simulink subsystem "HVACEmpiricalRef"  (R2024b)
settings: Solver=VariableStepAuto  StartTime=0.0  StopTime=10.0  RelTol=1e-3
undefined symbols (not defined in the file or in its folder): HVAC, vehicleThermal
libraries: fl_lib x70, nesl_utility x25, ee_lib x1
(part 1 of 2)
Description:
  | HVAC Empirical Reference
  | 
  | ⚡ Main Features:
  | - Empirical-based HVAC model with cabin and refrigeration subsystems
  | - Inputs: environment temperature, blower, PTC, compressor commands
  | - Refrigeration block models evaporator and compressor operation
  | - PTC heater and blower for cabin heating and airflow control
  | - Controlled current source represents HVAC electrical power draw
  | - Energy block tracks HVAC consumption from HV bus
  | 
  | 📤 Outputs: Cabin Temperature, HVAC Energy, Blower/Cooler/PTC States
  | 
  | 📌 Use Case: Fast empirical HVAC representation for cabin comfort and energy demand studies
settings Model: Creator=shachind  LastModifiedBy=jjha
settings RTWCC: GPUComputeCapability=3.5

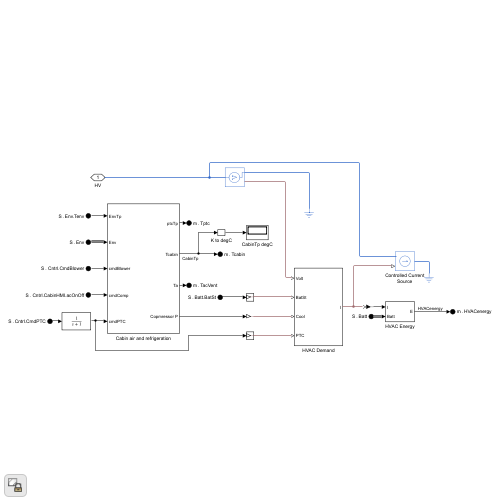
[thumbnail: Simulink's stored preview of the top-level diagram]
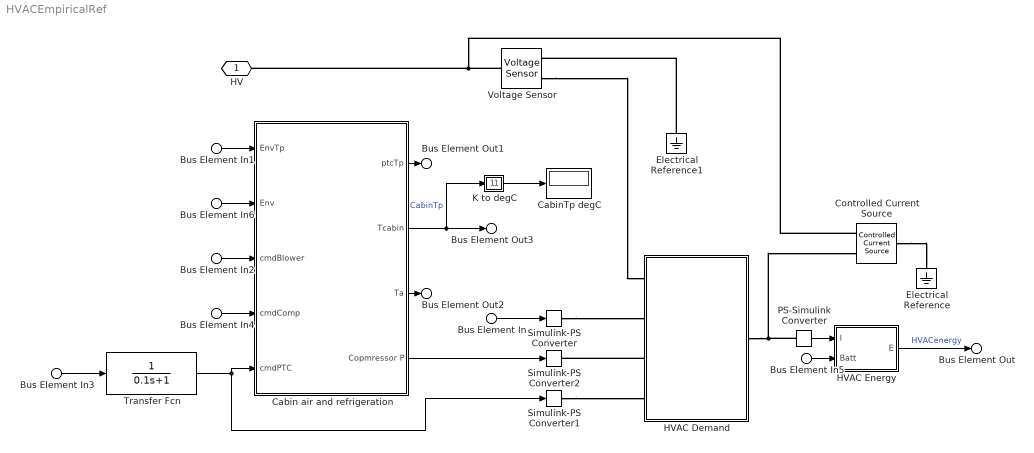
== system HVACEmpiricalRef ==
  Bus Element In5 : Inport  PortName=S  Element=Batt
  Bus Element In : Inport  PortName=S  Element=Batt.BatSt
  Bus Element In2 : Inport  PortName=S  Element=Cntrl.CmdBlower
  Bus Element In3 : Inport  PortName=S  Element=Cntrl.CmdPTC
  Bus Element In4 : Inport  PortName=S  Element=Cntrl.acOnOff
  Bus Element In6 : Inport  PortName=S  Element=Env
  Bus Element In1 : Inport  PortName=S  Element=Env.Tenv
  Cabin air and refrigeration : Subsystem
  CabinTp degC : Display
  Controlled Current Source : fl_lib/Electrical/Electrical Sources/Controlled Current Source
  Electrical Reference : fl_lib/Electrical/Electrical Elements/Electrical Reference
  Electrical Reference1 : fl_lib/Electrical/Electrical Elements/Electrical Reference
  HVAC Demand : Subsystem
  HVAC Energy : Subsystem
  K to degC : Subsystem
  PS-Simulink Converter : nesl_utility/PS-Simulink Converter  PhysicalDomain=network_engine_domain  SubClassName=ps_output  LeftPortType=input  RightPortType=output  PseudoPeriodic=off  Frequencies=[]  VectorFormat=inherit  Unit=inherit  AffineConversion=off
  Simulink-PS Converter : nesl_utility/Simulink-PS Converter  PhysicalDomain=network_engine_domain  SubClassName=ps_input  LeftPortType=input  RightPortType=output  PseudoPeriodic=off  Frequencies=[]  NoiseDistribution=none  NoiseParameters=[]  Unit=1  AffineConversion=off  FilteringAndDerivatives=provide  SimscapeFilterOrder=1  InputFilterTimeConstant=0.001  UdotUserProvided=0
  Simulink-PS Converter1 : nesl_utility/Simulink-PS Converter  PhysicalDomain=network_engine_domain  SubClassName=ps_input  LeftPortType=input  RightPortType=output  PseudoPeriodic=off  Frequencies=[]  NoiseDistribution=none  NoiseParameters=[]  Unit=W  AffineConversion=off  FilteringAndDerivatives=provide  SimscapeFilterOrder=1  InputFilterTimeConstant=0.001  UdotUserProvided=0
  Simulink-PS Converter2 : nesl_utility/Simulink-PS Converter  PhysicalDomain=network_engine_domain  SubClassName=ps_input  LeftPortType=input  RightPortType=output  PseudoPeriodic=off  Frequencies=[]  NoiseDistribution=none  NoiseParameters=[]  Unit=W  AffineConversion=off  FilteringAndDerivatives=provide  SimscapeFilterOrder=1  InputFilterTimeConstant=0.001  UdotUserProvided=0
  Transfer Fcn : TransferFcn  Denominator=[0.1 1]
  Voltage Sensor : fl_lib/Electrical/Electrical Sensors/Voltage Sensor
  HV : PMIOPort  Side=Left
  Bus Element Out : Outport  PortName=m  Element=HVACenergy
  Bus Element Out1 : Outport  PortName=m  Element=Tptc
  Bus Element Out3 : Outport  PortName=m  Element=Tcabin
  Bus Element Out2 : Outport  PortName=m  Element=TacVent
  wires:
  Bus Element In6/1 -> Cabin air and refrigeration/2(Env)
  Bus Element In2/1 -> Cabin air and refrigeration/3(cmdBlower)
  Cabin air and refrigeration/1(ptcTp) -> Bus Element Out1/1
  HVAC Energy/1(E) -> Bus Element Out/1  "HVACenergy"
  Bus Element In1/1 -> Cabin air and refrigeration/1(EnvTp)
  PS-Simulink Converter/1 -> HVAC Energy/1(I)
  Bus Element In5/1 -> HVAC Energy/2(Batt)
  Cabin air and refrigeration/4(Copmressor P) -> Simulink-PS Converter2/1
  Bus Element In3/1 -> Transfer Fcn/1
  Bus Element In/1 -> Simulink-PS Converter/1
  Cabin air and refrigeration/3(Ta) -> Bus Element Out2/1
  Bus Element In4/1 -> Cabin air and refrigeration/4(cmdComp)
  K to degC/1("  ") -> CabinTp degC/1
  Cabin air and refrigeration/2(Tcabin) -> K to degC/1(" "), Bus Element Out3/1  "CabinTp"
  Transfer Fcn/1 -> Simulink-PS Converter1/1, Cabin air and refrigeration/5(cmdPTC)
  connections:
  Controlled Current Source/RConn2 -- HV/RConn1 -- Voltage Sensor/LConn1
  PS-Simulink Converter/LConn1 -- Controlled Current Source/RConn1 -- HVAC Demand/RConn1
  Controlled Current Source/LConn1 -- Electrical Reference/LConn1
  Voltage Sensor/RConn1 -- HVAC Demand/LConn1
  Simulink-PS Converter/RConn1 -- HVAC Demand/LConn2
  HVAC Demand/LConn3 -- Simulink-PS Converter2/RConn1
  Simulink-PS Converter1/RConn1 -- HVAC Demand/LConn4
  Electrical Reference1/LConn1 -- Voltage Sensor/RConn2

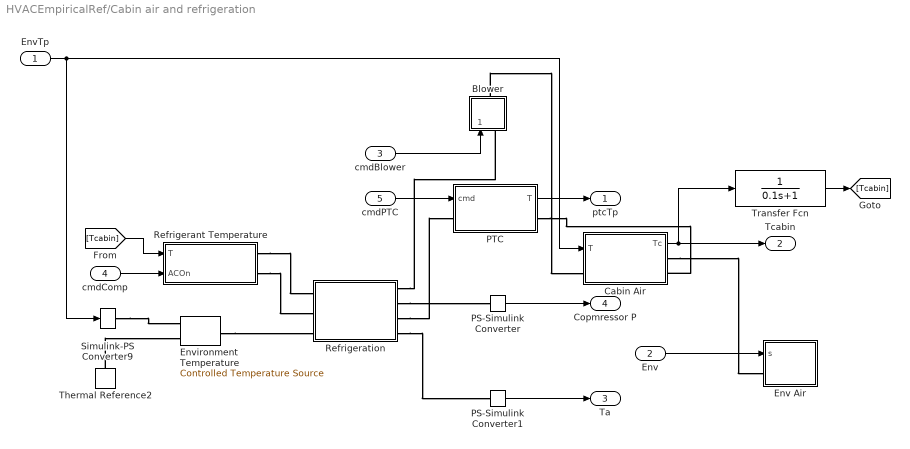
== system HVACEmpiricalRef/Cabin air and refrigeration ==
  EnvTp : Inport
  Env : Inport  Port=2
  cmdBlower : Inport  Port=3
  cmdComp : Inport  Port=4
  cmdPTC : Inport  Port=5
  Blower : Subsystem  Tag=PublishSubsystem
      mask Display:
      | plot(100*cos(linspace(0, 2*pi, 500)), 100*sin(linspace(0, 2*pi, 500)))
      | plot([28 80], [96 -60])
      | plot([-28 -80], [96 -60])
      | patch(-50*sin(3*linspace(0, pi, 500)).*cos(linspace(0, pi, 500)), -50*sin(3*linspace(0, pi, 500)).*sin(linspace(0, pi, 500)), [0 0 0])
  Cabin Air : Subsystem
      mask Display: disp(get_param(gcb, 'Name'))
  Env Air : Subsystem
  Environment Temperature : fl_lib/Thermal/Thermal Sources/Controlled Temperature Source
  PS-Simulink Converter : nesl_utility/PS-Simulink Converter  PhysicalDomain=network_engine_domain  SubClassName=ps_output  LeftPortType=input  RightPortType=output  PseudoPeriodic=off  Frequencies=[]  VectorFormat=inherit  Unit=inherit  AffineConversion=off
  PS-Simulink Converter1 : nesl_utility/PS-Simulink Converter  PhysicalDomain=network_engine_domain  SubClassName=ps_output  LeftPortType=input  RightPortType=output  PseudoPeriodic=off  Frequencies=[]  VectorFormat=inherit  Unit=inherit  AffineConversion=off
  PTC : Subsystem
      mask Display: disp(get_param(gcb, 'Name'))
  Refrigerant Temperature : Subsystem  mask{RefTemp=225.25}
      mask prompts: RefTemp "Condensor Refrigerant Temperature  [K]"
      mask DialogControl Refrigerant_temp Prompt: Parameters
  Refrigeration : Subsystem  mask{mRefEvap=1, mTubeEvap=1, tubeDiaEvap=0.01, tubeThickEvap=0.001, tubeLEvap=10, htcBoil=400, mRefCond=1, tubeDiaCond=0.01, tubeThickCond=0.001, tubeLCond=10, htcCondense=400, systemEfficiency=0.75}
      mask prompts: mRefEvap "Refrigerant mass inside evaporator (kg)"; mTubeEvap "Tube mass (kg)"; tubeDiaEvap "Tube outer diameter (m)"; tubeThickEvap "Tube wall thickness (m)"; tubeLEvap "Total length of the tube (m)"; htcBoil "Nucleate boiling HTC (W/K-m^2)"; mRefCond "Refrigerant mass inside Condensor (kg)"; tubeDiaCond "Tube outer diameter (m)"; tubeThickCond "Tube wall thickness (m)"; tubeLCond "Total length of the tube (m)"; htcCondense "Film condensation HTC (W/K-m^2)"; systemEfficiency "Overall system efficiency"
      mask DialogControl Container2 Prompt: Evaporator params
      mask DialogControl Container3 Prompt: Condensor params
      mask DialogControl Container4 Prompt: System params
      mask Display: disp(get_param(gcb, 'Name'))
  Simulink-PS Converter9 : nesl_utility/Simulink-PS Converter  PhysicalDomain=network_engine_domain  SubClassName=ps_input  LeftPortType=input  RightPortType=output  PseudoPeriodic=off  Frequencies=[]  NoiseDistribution=none  NoiseParameters=[]  Unit=K  AffineConversion=on  FilteringAndDerivatives=provide  SimscapeFilterOrder=1  InputFilterTimeConstant=0.001  UdotUserProvided=0
  Thermal Reference2 : fl_lib/Thermal/Thermal Elements/Thermal Reference
  Transfer Fcn : TransferFcn  Denominator=[0.1 1]
  ptcTp : Outport
  Tcabin : Outport  Port=2
  Ta : Outport  Port=3
  Copmressor P : Outport  Port=4
  wires:
  Transfer Fcn/1 -> [Tcabin]
  Env/1 -> Env Air/1(s)
  Cabin Air/1(Tc) -> Tcabin/1, Transfer Fcn/1
  PS-Simulink Converter1/1 -> Ta/1
  PS-Simulink Converter/1 -> Copmressor P/1
  PTC/1(T) -> ptcTp/1
  cmdBlower/1 -> Blower/1(cmd_blower)
  [Tcabin] -> Refrigerant Temperature/1(T)
  EnvTp/1 -> Simulink-PS Converter9/1, Cabin Air/1(T)
  cmdComp/1 -> Refrigerant Temperature/2(ACOn)
  cmdPTC/1 -> PTC/1(cmd)
  connections:
  Cabin Air/RConn1 -- Env Air/LConn1
  PTC/RConn1 -- Cabin Air/RConn2
  Blower/RConn1 -- Cabin Air/LConn1
  Refrigeration/RConn4 -- PS-Simulink Converter1/LConn1
  Refrigeration/RConn3 -- PTC/LConn1
  Refrigeration/RConn2 -- PS-Simulink Converter/LConn1
  Refrigeration/RConn1 -- Blower/LConn1
  Simulink-PS Converter9/RConn1 -- Environment Temperature/RConn1
  Environment Temperature/LConn1 -- Refrigeration/LConn3
  Thermal Reference2/LConn1 -- Environment Temperature/RConn2
  Refrigerant Temperature/RConn2 -- Refrigeration/LConn2
  Refrigerant Temperature/RConn1 -- Refrigeration/LConn1

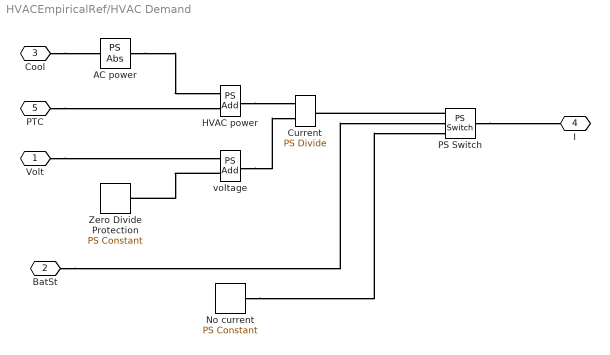
== system HVACEmpiricalRef/HVAC Demand ==
  AC power : fl_lib/Physical Signals/Nonlinear Operators/PS Abs
      settings: InternalSimscapePortConfiguration="{\"Bottom\":[],\"Left\":[{\"id\":\"I\",\"label\":\"\",\"type\":\"input\"}],\"Right\":[{\"id\":\"O\",\"label\":\"\",\"type\":\"output\"}],\"Top\":[]}"
  "Current " : fl_lib/Physical Signals/Functions/PS Divide
  HVAC power : fl_lib/Physical Signals/Functions/PS Add
  No current : fl_lib/Physical Signals/Sources/PS Constant  constant=0 A
  PS Switch : fl_lib/Physical Signals/Nonlinear Operators/PS Switch  Threshold=0.5
      settings: InternalSimscapePortConfiguration="{\"Bottom\":[],\"Left\":[{\"id\":\"I1\",\"label\":\"\",\"type\":\"input\"},{\"id\":\"I2\",\"label\":\"\",\"type\":\"input\"},{\"id\":\"I3\",\"label\":\"\",\"type\":\"input\"}],\"Right\":[{\"id\":\"O\",\"label\":\"\",\"type\":\"output\"}],\"Top\":[]}"
  Zero Divide Protection : fl_lib/Physical Signals/Sources/PS Constant  constant=10 V
  voltage : fl_lib/Physical Signals/Functions/PS Add
  Volt : PMIOPort  Side=Left
  BatSt : PMIOPort  Port=2  Side=Left
  Cool : PMIOPort  Port=3  Side=Left
  I : PMIOPort  Port=4  Side=Right
  PTC : PMIOPort  Port=5  Side=Left
  connections:
  Volt/RConn1 -- voltage/LConn1
  HVAC power/RConn1 -- "Current "/LConn1
  PTC/RConn1 -- HVAC power/LConn2
  Cool/RConn1 -- AC power/LConn1
  AC power/RConn1 -- HVAC power/LConn1
  voltage/LConn2 -- Zero Divide Protection/RConn1
  voltage/RConn1 -- "Current "/LConn2
  PS Switch/RConn1 -- I/RConn1
  BatSt/RConn1 -- PS Switch/LConn2
  PS Switch/LConn1 -- "Current "/RConn1
  No current/RConn1 -- PS Switch/LConn3

== system HVACEmpiricalRef/HVAC Energy ==
  I : Inport
  Batt : Inport  Port=2
  Bus Selector : BusSelector  OutputSignals=BattSensor.BatVolt
  Constant : Constant  Value=3600
  Divide : Product  Inputs=*/
  Integrator : Integrator
  Product : Product
  E : Outport
  wires:
  Bus Selector/1 -> Product/2  "<BatVolt>"
  Product/1 -> Integrator/1
  Integrator/1 -> Divide/1
  Constant/1 -> Divide/2
  Batt/1 -> Bus Selector/1
  Divide/1 -> E/1
  I/1 -> Product/1

== system HVACEmpiricalRef/K to degC ==
  " " : Inport
  Constant : Constant  Value=273.15
  Subtract : Sum  Inputs=+-
  "  " : Outport
  wires:
  Constant/1 -> Subtract/2
  Subtract/1 -> "  "/1
  " "/1 -> Subtract/1

== system HVACEmpiricalRef/Cabin air and refrigeration/Blower ==
  cmd_blower : Inport
  Blower : fl_lib/Moist Air/Sources/Flow Rate Source (MA)  source_type=foundation.enum.constant_controlled.controlled  flow_type=foundation.enum.mass_volumetric_flow.volumetric  mass_flow=0 kg/s  volumetric_flow=0 m^3/s  volumetric_flow_conditions=foundation.enum.volumetric_flow_conditions.standard  p_std=0.101325 MPa  T_std=vehicleThermal.cabin_T_init K  RH_std=0.65  power_spec=foundation.enum.power_spec.isentropic  area_A=HVAC.cabin_duct_area m^2  area_B=HVAC.cabin_duct_area m^2
      settings: InternalSimscapePortConfiguration="{\"Bottom\":[],\"Left\":[{\"id\":\"A\",\"label\":\"A\",\"type\":\"foundation.moist_air.moist_air\"},{\"id\":\"V\",\"label\":\"V\",\"type\":\"input\"}],\"Right\":[{\"id\":\"B\",\"label\":\"B\",\"type\":\"foundation.moist_air.moist_air\"}],\"Top\":[]}"
  Max Flow [m^3/s] : Gain  Gain=0.15
  Moist Air Properties : fl_lib/Moist Air/Utilities/Moist Air Properties (MA)  R_a=287.047 J/kg/K  T_TLU=[-56.55, -50 : 10 : -10, -5 : 1 : 5, 10 : 10 : 350]' degC  h_a_TLU=[342.416126230579; 349.005511058471; 359.063577249119; 369.119948684177; 379.175469465129; 389.230944678417; 394.258910928084; 395.264534937366; 396.27017101329; 397.275819932805; 398.281482472874; 399.287159410541; 400.292851523015; 401.298559587728; 402.304284382408; 403.310026685143; 404.315787274435; 409.34489180313; 419.404921755863; 429.468036401264; 439.535033154839; 449.606720928652; 459.683919949603; 469.767460521911; 479.858181001348; 489.956925196484; 500.064539372946; 510.181869006204; 520.309755403634; 530.449032296018; 540.60052248087; 550.765034584465; 560.943359995745; 571.136270013102; 581.344513234296; 591.568813210327; 601.809866375885; 612.068340261954; 622.344871990218; 632.640067043998; 642.95449830646; 653.288705353699; 663.643193987949; 674.018435994423; 684.414869104228; 694.832897145098; 705.272890361557; 715.735185886199; 726.220088344236; 736.727870574087; 747.258774447567; 757.813011774199] kJ/kg  mu_a_TLU=[14.2568883320012; 14.6140127728333; 15.1517277055779; 15.6806860159119; 16.2012351072083; 16.7137043125028; 16.9670071730589; 17.017438062815; 17.0677930842452; 17.1180725309876; 17.1682766951315; 17.2184058672268; 17.2684603362935; 17.3184403898301; 17.3683463138234; 17.4181783927569; 17.4679369096204; 17.7156358640698; 18.2056751785154; 18.68879035749; 19.1652344664982; 19.6352478927873; 20.099059103658; 20.5568853601578; 21.0089333871663; 21.4554000014051; 21.8964726992323; 22.3323302062775; 22.7631429910631; 23.1890737447833; 23.6102778293792; 24.0269036959922; 24.4390932757886; 24.8469823450548; 25.2507008663546; 25.6503733074314; 26.0461189394339; 26.4380521159325; 26.8262825340948; 27.2109154792923; 27.5920520543128; 27.969789394274; 28.3442208682439; 28.7154362685068; 29.0835219883356; 29.4485611890712; 29.8106339572472; 30.1698174524429; 30.5261860464955; 30.8798114546565; 31.2307628592324; 31.5791070262086] s*uPa  k_a_TLU=[19.8808489374933; 20.4162454629695; 21.2248743590758; 22.0232452890903; 22.8117314495857; 23.5906913619588; 23.9767075412237; 24.053639990175; 24.1304826682191; 24.2072359051629; 24.2839000294007; 24.3604753679152; 24.4369622462801; 24.5133609886625; 24.5896719178249; 24.6658953551279; 24.7420316205333; 25.1214164701832; 25.8738283029331; 26.6180150229276; 27.3542674377332; 28.0828634735341; 28.8040686837224; 29.5181367785657; 30.2253101618423; 30.9258204644224; 31.6198890677835; 32.3077276126633; 32.9895384896798; 33.6655153099498; 34.33584335461; 35.0007000027879; 35.6602551380254; 36.3146715334901; 36.9641052165342; 37.6087058133173; 38.248616874307; 38.8839761815308; 39.5149160384798; 40.1415635435708; 40.7640408480637; 41.3824653993118; 41.9969501701893; 42.6076038755117; 43.2145311762238; 43.8178328720941; 44.4176060836121; 45.013944423749; 45.6069381602018; 46.1966743687041; 46.783237077953; 47.3667074066625] mW/m/K  p_min=1 kPa  p_max=inf MPa  T_min=-56.55 degC  T_max=350 degC  properties_range_check=simscape.enum.assert.action.error  p_atm=0.101325 MPa  T_atm=vehicleThermal.cabin_T_init K  enable_droplets=false  R_w=461.523 J/kg/K  p_ws_TLU=[1.71168953425982e-06; 3.93770601979424e-06; 1.28411717710344e-05; 3.80051394873809e-05; .00010323902900209; .000259873810798063; .000401741022116384; .000437454836117844; .000476040820618202; .000517704666185737; .000562664883741207; .000611212677444345; .000657088049117899; .000705987905898279; .000758082381149132; .000813549384183233; .000872574861129522; .00122818386934022; .0023392147667769; .00424668834054807; .00738442748706953; .0123512704340234; .0199458019246787; .0312006356960619; .0474147199263783; .0701823607447713; .10141797792131; .143375967241115; .198665399739302; .270259606559999; .361500961984849; .476101381081492; .618139196722055; .792053183687694; 1.0026345688121; 1.25501792086105; 1.55467186826983; 1.90739066433297; 2.31928772772542; 2.79679245576864; 3.34665187151016; 3.97593907083533; 4.69207105435535; 5.5028394740883; 6.41645928168037; 7.4416425436169; 8.58770832955728; 9.86474556030261; 11.2838558865497; 12.8575218898034; 14.6001810568052; 16.5291642526045] MPa  h_w_vap_TLU=[2836.88241275372; 2837.81392500514; 2838.63937175807; 2838.7309929628; 2838.06905313927; 2836.62597341095; 2835.60023952573; 2835.37006381376; 2835.13143158077; 2834.88429145066; 2834.62859062897; 2500.93420564316; 2498.55329907119; 2496.17495082036; 2493.79885912205; 2491.42474723191; 2489.05236104642; 2477.20875029194; 2453.54955988604; 2429.83856603313; 2406.00136954922; 2381.97406342174; 2357.69101156389; 2333.08088387814; 2308.06565480412; 2282.56034405021; 2256.47287422313; 2229.70428017508; 2202.14968030993; 2173.69998896199; 2144.24368406447; 2113.66758247452; 2081.85585110571; 2048.68725710494; 2014.03141249899; 1977.7449923284; 1939.66849592886; 1899.62342931686; 1857.40930169838; 1812.79975416601; 1765.53721731251; 1715.32525772152; 1661.81700477787; 1604.59703745016; 1543.1534616334; 1476.83692476464; 1404.80240352424; 1325.92091736114; 1238.61667822208; 1140.5102987018; 1027.62017777647; 892.733785613825] kJ/kg  h_w_TLU=[2396.55944251649; 2408.68643343608; 2427.1988031141; 2445.702165897; 2464.18429108356; 2482.62529466839; 2491.82135326629; 2493.6580151792; 2495.49372578218; 2497.32843835745; 2499.16210446923; 2500.99462758899; 2502.83092214066; 2504.6665223621; 2506.50140563013; 2508.335548891; 2510.16892865793; 2519.32352241995; 2537.56068088674; 2555.67742615292; 2573.6403223998; 2591.4109179101; 2608.9455037701; 2626.19492016262; 2643.10444358428; 2659.61377634497; 2675.58278696023; 2696.1846256545; 2716.49989553741; 2736.6235210957; 2756.61216047011; 2776.50561773853; 2796.33378922508; 2816.11979583049; 2835.88181423877; 2855.63430574511; 2875.38889327595; 2895.15500577172; 2914.94035964689; 2934.75132290228; 2954.59319330244; 2974.47041285505; 2994.38673458964; 3014.34535328009; 3034.34900867103; 3054.40006755764; 3074.50058946898; 3094.65237953784; 3114.85703128106; 3135.11596137801; 3155.43043805905; 3175.80160435813] kJ/kg  mu_w_TLU=[6.81365662228272; 7.04953750742707; 7.40970098298307; 7.76991278093907; 8.13017290129507; 8.49048134405107; 8.67065368632907; 8.70668960445667; 8.74272600580827; 8.77876289038387; 8.81480025818347; 8.85083810920707; 8.88687644345467; 8.92291526092627; 8.95895456162187; 8.99499434554147; 9.03103461268507; 9.21124319676307; 9.57169660671907; 9.93219833907507; 10.2927483938311; 10.6533467709871; 11.0139934705431; 11.3746884924991; 11.7354318368551; 12.0962235036111; 12.4570634927671; 12.8179518043231; 13.1788884382791; 13.5398733946351; 13.9009066733911; 14.2619882745471; 14.6231181981031; 14.9842964440591; 15.3455230124151; 15.7067979031711; 16.0681211163271; 16.4294926518831; 16.7909125098391; 17.1523806901951; 17.5138971929511; 17.8754620181071; 18.2370751656631; 18.5987366356191; 18.9604464279751; 19.3222045427311; 19.6840109798871; 20.0458657394431; 20.4077688213991; 20.7697202257551; 21.1317199525111; 21.4937680016671] s*uPa  k_w_TLU=[11.46288215976; 11.941997488935; 12.676358586935; 13.414208884935; 14.155548382935; 14.900377080935; 15.274099879935; 15.348949115735; 15.423833243535; 15.498752263335; 15.573706175135; 15.648694978935; 15.723718674735; 15.798777262535; 15.873870742335; 15.948999114135; 16.024162377935; 16.400502076935; 17.155798374935; 17.914583872935; 18.676858570935; 19.442622468935; 20.211875566935; 20.984617864935; 21.760849362935; 22.540570060935; 23.323779958935; 24.110479056935; 24.900667354935; 25.694344852935; 26.491511550935; 27.292167448935; 28.096312546935; 28.903946844935; 29.715070342935; 30.529683040935; 31.347784938935; 32.169376036935; 32.994456334935; 33.823025832935; 34.655084530935; 35.490632428935; 36.329669526935; 37.172195824935; 38.018211322935; 38.867716020935; 39.720709918935; 40.577193016935; 41.437165314935; 42.300626812935; 43.167577510935; 44.038017408935] mW/m/K  D_w=25 mm^2/s  trace_gas_model=foundation.enum.trace_gas_model.track_fraction  R_g=188.923 J/kg/K  h_g_TLU=[439.555216260064; 444.670268200251; 452.538618847003; 460.487124258496; 468.522588768941; 476.649415958793; 480.74798538725; 481.57054318762; 482.394052398751; 483.218514288831; 484.043930029015; 484.870300696555; 485.697627277859; 486.525910671489; 487.355151691079; 488.185351068185; 489.016509455051; 493.186704139431; 501.599194953048; 510.107689961685; 518.711611080182; 527.410026793075; 536.201764778798; 545.085474203452; 554.059675505208; 563.122805485367; 572.27325096919; 581.509373027928; 590.829525105886; 600.232066705818; 609.715373581392; 619.277845178105; 628.917909922924; 638.634028838794; 648.424697859328; 658.288449140109; 668.223851601449; 678.229510889093; 688.304068901113; 698.44620299875; 708.654624994591; 718.928079991818; 729.265345132425; 739.665228299475; 750.126566808087; 760.648226111439; 771.229098541268; 781.868102096908; 792.564179292476; 803.316296068366; 814.123440770426; 824.984623198037] kJ/kg  mu_g_TLU=[10.8921054191698; 11.2215357085649; 11.7233300740382; 12.2234238147811; 12.7215124453467; 13.2173328890673; 13.4643203184773; 13.5136406274989; 13.562934752385; 13.6122025024997; 13.6614436900741; 13.7106581301692; 13.7598456406398; 13.8090060420983; 13.8581391578796; 13.9072448140062; 13.9563228391538; 14.2012926853717; 14.6890687376044; 15.1738428124161; 15.6554929043332; 16.1339159800463; 16.6090257998657; 17.0807510097148; 17.5490334645512; 18.0138267508952; 18.4750948814453; 18.9328111390399; 19.3869570507278; 19.8375214755778; 20.2844997922255; 20.7278931741254; 21.1677079421287; 21.6039549853963; 22.036649242835; 22.4658092382469; 22.8914566632375; 23.3136160026627; 23.7323141980278; 24.1475803447965; 24.5594454200432; 24.9679420372927; 25.3731042257492; 25.774967231431; 26.1735673380029; 26.5689417053362; 26.9611282240413; 27.350165384404; 27.73609215832; 28.118947892972; 28.4987722151178; 28.8756049449796] s*uPa  k_g_TLU=[10.489430678843; 10.9507672150864; 11.666197960308; 12.392559739764; 13.1299519771612; 13.8778409888416; 14.2554325416312; 14.3312274189707; 14.4071122346908; 14.4830860227061; 14.5591478179508; 14.6352966574703; 14.7115315815553; 14.787851634907; 14.8642558678259; 14.9407433374142; 15.0173131087819; 15.401364480906; 16.1751373988038; 16.9558134611595; 17.7432208682398; 18.5366976599676; 19.3360988502003; 20.1412225692689; 20.9517507672929; 21.7672310558863; 22.5871115634685; 23.4107980865695; 24.2377021890869; 25.0672663781241; 25.8989689893876; 26.732318357514; 27.5668446164644; 28.4020933015927; 29.2376215872816; 30.0729965057542; 30.9077942826816; 31.7416001931033; 32.5740086297993; 33.4046232539953; 34.2330571812868; 35.0589331874899; 35.8818839295189; 36.701552179391; 37.5175910702657; 38.3296643536716; 39.1374466671854; 39.9406238119064; 40.7388930391313; 41.5319633456945; 42.3195557774861; 43.1014037407076] mW/m/K  D_g=16 mm^2/s
  Simulink-PS Converter : nesl_utility/Simulink-PS Converter  PhysicalDomain=network_engine_domain  SubClassName=ps_input  LeftPortType=input  RightPortType=output  PseudoPeriodic=off  Frequencies=[]  NoiseDistribution=none  NoiseParameters=[]  Unit=m^3/s  AffineConversion=off  FilteringAndDerivatives=provide  SimscapeFilterOrder=1  InputFilterTimeConstant=0.001  UdotUserProvided=0
  Transfer Fcn : TransferFcn  Denominator=[5 1]
  B : PMIOPort  Side=Left
  A : PMIOPort  Port=2  Side=Right
  wires:
  Max Flow [m^3/s]/1 -> Simulink-PS Converter/1
  Transfer Fcn/1 -> Max Flow [m^3/s]/1
  cmd_blower/1 -> Transfer Fcn/1
  connections:
  Blower/RConn1 -- B/RConn1
  Blower/LConn2 -- Simulink-PS Converter/RConn1
  A/RConn1 -- Blower/LConn1 -- Moist Air Properties/RConn1

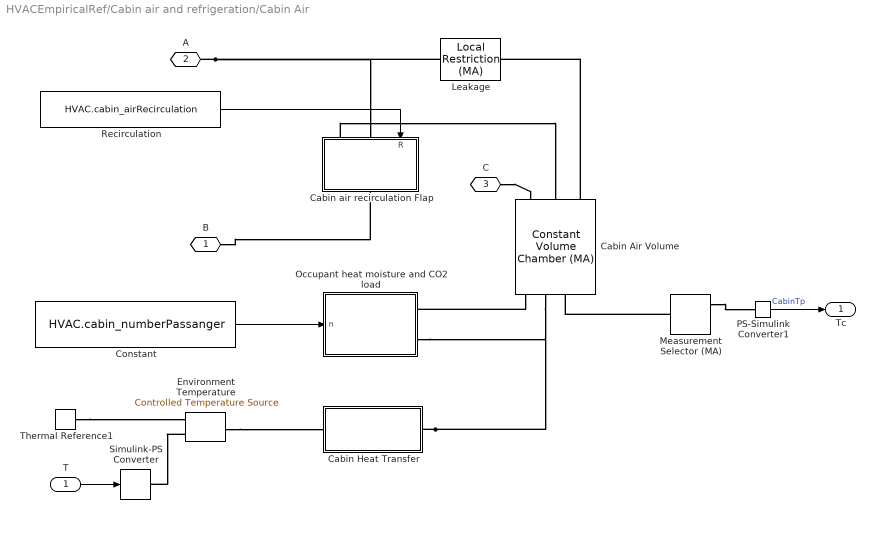
== system HVACEmpiricalRef/Cabin air and refrigeration/Cabin Air ==
  T : Inport
  Cabin Air Volume : fl_lib/Moist Air/Elements/Constant Volume Chamber (MA)  volume=3 m^3  num_ports=foundation.enum.num_ports.three  area_A=1 m^2  area_B=HVAC.cabin_duct_area m^2  area_C=HVAC.cabin_duct_area m^2  area_D=0.01 m^2  RH_ws=1  time_constant_cond=1e-3 s  time_constant_evap=1e-3 s  fraction_entrained=1  moisture_trace_gas_source=foundation.enum.moisture_trace_gas_source.controlled  moisture_source_spec=foundation.enum.MoistureSourceSpec.WaterVapor  vapor_from_liquid=false  moisture_mass_flow=0 kg/s  moisture_temperature_spec=foundation.enum.temperature_spec.atmospheric  moisture_temperature=293.15 K  trace_gas_mass_flow=0 kg/s  trace_gas_temperature_spec=foundation.enum.temperature_spec.atmospheric  trace_gas_temperature=293.15 K  p_init=vehicleThermal.cabin_p_init MPa  p_init_priority=foundation.enum.Priority.High  T_init=vehicleThermal.cabin_T_init K  T_init_priority=foundation.enum.Priority.High  humidity_spec=foundation.enum.HumiditySpec.RelativeHumidity  RH_init=vehicleThermal.cabin_RH_init  RH_init_priority=foundation.enum.Priority.High  x_w_init=0  x_w_init_priority=foundation.enum.Priority.None  y_w_init=0  y_w_init_priority=foundation.enum.Priority.None  HR_init=0  HR_init_priority=foundation.enum.Priority.None  Tw_init=287 K  Tw_init_priority=foundation.enum.Priority.High  trace_gas_spec=foundation.enum.trace_gas_spec.mass_fraction  x_g_init=0  x_g_init_priority=foundation.enum.Priority.High  y_g_init=0  y_g_init_priority=foundation.enum.Priority.None  r_d_init=0  r_d_init_priority=foundation.enum.Priority.High
      settings: InternalSimscapePortConfiguration="{\"Bottom\":[],\"Left\":[{\"id\":\"A\",\"label\":\"A\",\"type\":\"foundation.moist_air.moist_air\"},{\"id\":\"B\",\"label\":\"B\",\"type\":\"foundation.moist_air.moist_air\"},{\"id\":\"C\",\"label\":\"C\",\"type\":\"foundation.moist_air.moist_air\"}],\"Right\":[{\"id\":\"W\",\"label\":\"W\",\"type\":\"output\"},{\"id\":\"F\",\"label\":\"F\",\"type\":\"output\"},{\"id\":\"H\",\"label\":\"H\",\"type\":\"foundation.thermal.thermal\"},{\"id\":\"S\",\"label\":\"S\",\"type\":\"foundation.moist_air.moist_air_source\"}],\"Top\":[]}"
  Cabin Heat Transfer : Subsystem  Tag=PublishSubsystem  mask(Cabin Heat Transfer){glass_area=3.5, glass_thickness=0.004, glass_mass=3.5 * 0.004 * 2600, glass_specific_heat=840, glass_conductivity=0.96, glass_heat_coeff=40, glass_initial_temperature=vehicleThermal.ambient, doors_area=4, doors_thickness=0.06, doors_mass=75, doors_specific_heat=500, doors_conductivity=0.08, doors_heat_coeff=40, doors_initial_temperature=vehicleThermal.ambient, roof_area=2, roof_thickness=0.04, roof_mass=30, roof_specific_heat=500, roof_conductivity=0.08, roof_heat_coeff=40, roof_initial_temperature=vehicleThermal.ambient}
      mask prompts: glass_area "Area (m^2)"; glass_thickness "Thickness (m)"; glass_mass "Mass (kg)"; glass_specific_heat "Specific heat (J/kg/K)"; glass_conductivity "Thermal conductivity (W/m/K)"; glass_heat_coeff "Convective heat transfer coefficient (W/m^2/K)"; glass_initial_temperature "Initial temperature (K)"; doors_area "Area (m^2)"; doors_thickness "Thickness (m)"; doors_mass "Mass (kg)"; doors_specific_heat "Specific heat (J/kg/K)"; doors_conductivity "Thermal conductivity (W/m/K)"; doors_heat_coeff "Convective heat transfer coefficient (W/m^2/K)"; doors_initial_temperature "Initial temperature (K)"; roof_area "Area (m^2)"; roof_thickness "Thickness (m)"; roof_mass "Mass (kg)"; roof_specific_heat "Specific heat (J/kg/K)"; roof_conductivity "Thermal conductivity (W/m/K)"; roof_heat_coeff "Convective heat transfer coefficient (W/m^2/K)"; roof_initial_temperature "Initial temperature (K)"
      mask DialogControl GlassTabVar Prompt: Glass
      mask DialogControl DoorsTabVar Prompt: Doors
      mask DialogControl RoofTabVar Prompt: Roof
  Cabin air recirculation Flap : Subsystem  Tag=PublishSubsystem  mask{min_area=1e-8 * HVAC.cabin_duct_area, max_area=0.9 *HVAC.cabin_duct_area, port_area=HVAC.cabin_duct_area, Cd=0.8, tau=1}
      mask prompts: min_area "Min restriction area (m^2)"; max_area "Max restriction area (m^2)"; port_area "Cross-sectional area at ports A, B, and C (m^2)"; Cd "Discharge coefficient"; tau "Opening time constant (s)"
  Constant : Constant  Value=HVAC.cabin_numberPassanger
  Environment Temperature : fl_lib/Thermal/Thermal Sources/Controlled Temperature Source
  Leakage : fl_lib/Moist Air/Elements/Local Restriction (MA)  restriction_type=foundation.enum.restriction_type.fixed  restriction_area=0.004 m^2  min_area=1e-10 m^2  max_area=0.005 m^2  area=1 m^2  Cd=0.8  B_lam=0.999
      settings: InternalSimscapePortConfiguration="{\"Bottom\":[],\"Left\":[{\"id\":\"A\",\"label\":\"A\",\"type\":\"foundation.moist_air.moist_air\"}],\"Right\":[{\"id\":\"B\",\"label\":\"B\",\"type\":\"foundation.moist_air.moist_air\"}],\"Top\":[]}"
  Measurement Selector (MA) : fl_lib/Moist Air/Sensors/Measurement Selector (MA)  moisture_spec=foundation.enum.moisture_spec.relative_humidity  trace_gas_spec=foundation.enum.trace_gas_spec.mass_fraction
      settings: InternalSimscapePortConfiguration="{\"Bottom\":[],\"Left\":[{\"id\":\"F\",\"label\":\"F\",\"type\":\"input\"}],\"Right\":[{\"id\":\"P\",\"label\":\"P\",\"type\":\"output\"},{\"id\":\"T\",\"label\":\"T\",\"type\":\"output\"},{\"id\":\"W\",\"label\":\"W\",\"type\":\"output\"},{\"id\":\"G\",\"label\":\"G\",\"type\":\"output\"},{\"id\":\"D\",\"label\":\"D\",\"type\":\"output\"}],\"Top\":[]}"
  Occupant heat moisture and CO2 load : Subsystem
  PS-Simulink Converter1 : nesl_utility/PS-Simulink Converter  PhysicalDomain=network_engine_domain  SubClassName=ps_output  LeftPortType=input  RightPortType=output  PseudoPeriodic=off  Frequencies=[]  VectorFormat=1-D array  Unit=K  AffineConversion=on
  Recirculation : Constant  Value=HVAC.cabin_airRecirculation
  Simulink-PS Converter : nesl_utility/Simulink-PS Converter  PhysicalDomain=network_engine_domain  SubClassName=ps_input  LeftPortType=input  RightPortType=output  PseudoPeriodic=off  Frequencies=[]  NoiseDistribution=none  NoiseParameters=[]  Unit=K  AffineConversion=on  FilteringAndDerivatives=provide  SimscapeFilterOrder=1  InputFilterTimeConstant=0.001  UdotUserProvided=0
  Thermal Reference1 : fl_lib/Thermal/Thermal Elements/Thermal Reference
  B : PMIOPort  Side=Left
  A : PMIOPort  Port=2  Side=Right
  C : PMIOPort  Port=3  Side=Right
  Tc : Outport
  wires:
  Constant/1 -> Occupant heat moisture and CO2 load/1(n)
  Recirculation/1 -> Cabin air recirculation Flap/1(R)
  T/1 -> Simulink-PS Converter/1
  PS-Simulink Converter1/1 -> Tc/1  "CabinTp"
  connections:
  Cabin Air Volume/RConn4 -- Occupant heat moisture and CO2 load/RConn1
  A/RConn1 -- Cabin air recirculation Flap/LConn1 -- Leakage/LConn1
  Cabin Air Volume/LConn1 -- Leakage/RConn1
  Cabin air recirculation Flap/LConn2 -- Cabin Air Volume/LConn2
  B/RConn1 -- Cabin air recirculation Flap/RConn1
  Cabin Heat Transfer/LConn1 -- Cabin Air Volume/RConn3 -- Occupant heat moisture and CO2 load/RConn2
  Environment Temperature/RConn1 -- Simulink-PS Converter/RConn1
  Thermal Reference1/LConn1 -- Environment Temperature/RConn2
  Environment Temperature/LConn1 -- Cabin Heat Transfer/RConn1
  C/RConn1 -- Cabin Air Volume/LConn3
  Measurement Selector (MA)/LConn1 -- Cabin Air Volume/RConn2
  Measurement Selector (MA)/RConn2 -- PS-Simulink Converter1/LConn1

== system HVACEmpiricalRef/Cabin air and refrigeration/Env Air ==
  s : Inport
  Environment Air : fl_lib/Moist Air/Elements/Reservoir (MA)  pressure_input=true  pressure_spec=foundation.enum.pressure_spec.atmospheric  reservoir_pressure=0.101325 MPa  temperature_input=true  temperature_spec=foundation.enum.temperature_spec.atmospheric  reservoir_temperature=293.15 K  humidity_input=true  humidity_spec=foundation.enum.HumiditySpec.RelativeHumidity  reservoir_RH=0.5  reservoir_x_w=0.01  reservoir_y_w=0.01  reservoir_HR=0.01  reservoir_Tw=287 K  trace_gas_input=true  trace_gas_spec=foundation.enum.trace_gas_spec.mole_fraction  reservoir_x_g=0.001  reservoir_y_g=0.001  water_droplets_input=false  reservoir_r_d=0  RH_ws=1  area_A=1 m^2  input_error_spec=foundation.enum.input_range_error.warn
      settings: InternalSimscapePortConfiguration="{\"Bottom\":[],\"Left\":[{\"id\":\"A\",\"label\":\"A\",\"type\":\"foundation.moist_air.moist_air\"}],\"Right\":[{\"id\":\"T\",\"label\":\"T\",\"type\":\"input\"},{\"id\":\"P\",\"label\":\"P\",\"type\":\"input\"},{\"id\":\"W\",\"label\":\"W\",\"type\":\"input\"},{\"id\":\"G\",\"label\":\"G\",\"type\":\"input\"}],\"Top\":[]}"
  Simulink-PS Converter1 : nesl_utility/Simulink-PS Converter  PhysicalDomain=network_engine_domain  SubClassName=ps_input  LeftPortType=input  RightPortType=output  PseudoPeriodic=off  Frequencies=[]  NoiseDistribution=none  NoiseParameters=[]  Unit=K  AffineConversion=on  FilteringAndDerivatives=provide  SimscapeFilterOrder=1  InputFilterTimeConstant=0.001  UdotUserProvided=0
  Simulink-PS Converter2 : nesl_utility/Simulink-PS Converter  PhysicalDomain=network_engine_domain  SubClassName=ps_input  LeftPortType=input  RightPortType=output  PseudoPeriodic=off  Frequencies=[]  NoiseDistribution=none  NoiseParameters=[]  Unit=MPa  AffineConversion=off  FilteringAndDerivatives=provide  SimscapeFilterOrder=1  InputFilterTimeConstant=0.001  UdotUserProvided=0
  Simulink-PS Converter3 : nesl_utility/Simulink-PS Converter  PhysicalDomain=network_engine_domain  SubClassName=ps_input  LeftPortType=input  RightPortType=output  PseudoPeriodic=off  Frequencies=[]  NoiseDistribution=none  NoiseParameters=[]  Unit=1  AffineConversion=off  FilteringAndDerivatives=provide  SimscapeFilterOrder=1  InputFilterTimeConstant=0.001  UdotUserProvided=0
  Simulink-PS Converter4 : nesl_utility/Simulink-PS Converter  PhysicalDomain=network_engine_domain  SubClassName=ps_input  LeftPortType=input  RightPortType=output  PseudoPeriodic=off  Frequencies=[]  NoiseDistribution=none  NoiseParameters=[]  Unit=1  AffineConversion=off  FilteringAndDerivatives=provide  SimscapeFilterOrder=1  InputFilterTimeConstant=0.001  UdotUserProvided=0
  Subsystem : Subsystem
  A : PMIOPort  Side=Left
  wires:
  Subsystem/2(p) -> Simulink-PS Converter2/1
  Subsystem/1(T) -> Simulink-PS Converter1/1
  s/1 -> Subsystem/1(s)
  Subsystem/4(CO2) -> Simulink-PS Converter4/1
  Subsystem/3(RH) -> Simulink-PS Converter3/1
  connections:
  A/RConn1 -- Environment Air/LConn1
  Simulink-PS Converter4/RConn1 -- Environment Air/RConn4
  Simulink-PS Converter1/RConn1 -- Environment Air/RConn1
  Simulink-PS Converter2/RConn1 -- Environment Air/RConn2
  Simulink-PS Converter3/RConn1 -- Environment Air/RConn3

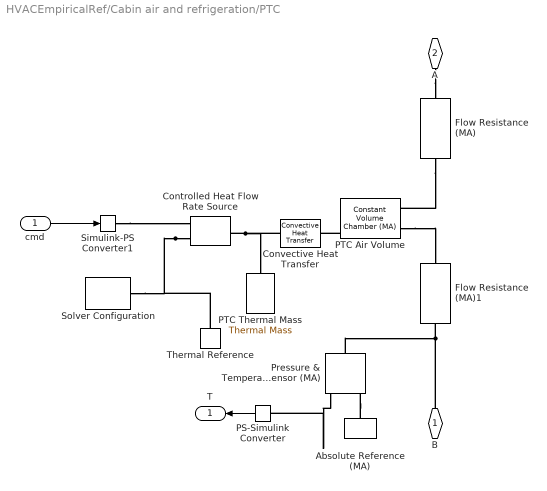
== system HVACEmpiricalRef/Cabin air and refrigeration/PTC ==
  cmd : Inport
  Absolute Reference (MA) : fl_lib/Moist Air/Elements/Absolute Reference (MA)
  Controlled Heat Flow Rate Source : fl_lib/Thermal/Thermal Sources/Controlled Heat Flow Rate Source
  Convective Heat Transfer : fl_lib/Thermal/Thermal Elements/Convective Heat Transfer  thermal_type=foundation.enum.constant_variable.constant  area=1 m^2  heat_tr_coeff=200 W/(m^2 * K)  min_heat_tr_coeff=1e-3 W/(K*m^2)  T_specify=off  T_priority=None  T=0 K  T_nominal_specify=off  T_nominal_value=cabin_T_init  T_nominal_unit=degC  Q_specify=off  Q_priority=None  Q=0 W  Q_nominal_specify=off  Q_nominal_value=1  Q_nominal_unit=W
  Flow Resistance (MA) : fl_lib/Moist Air/Elements/Flow Resistance (MA)  delta_p_nominal=2e-4 MPa  mdot_nominal=0.15 kg/s  rho_nominal=1.2 kg/m^3  area=HVAC.cabin_duct_area m^2  laminar_fraction=1e-3
  Flow Resistance (MA)1 : fl_lib/Moist Air/Elements/Flow Resistance (MA)  delta_p_nominal=2e-4 MPa  mdot_nominal=0.15 kg/s  rho_nominal=1.2 kg/m^3  area=HVAC.cabin_duct_area m^2  laminar_fraction=1e-3
  PS-Simulink Converter : nesl_utility/PS-Simulink Converter  PhysicalDomain=network_engine_domain  SubClassName=ps_output  LeftPortType=input  RightPortType=output  PseudoPeriodic=off  Frequencies=[]  VectorFormat=1-D array  Unit=K  AffineConversion=on
  PTC Thermal Mass : fl_lib/Thermal/Thermal Elements/Thermal Mass  mass_type=foundation.enum.constant_variable.constant  mass=1.5 kg  sp_heat=447 J/(K*kg)  mass_min=1e-6 kg  num_ports=foundation.enum.numPorts2.one  m_specify=off  m_priority=High  m=1 kg  m_nominal_specify=off  m_nominal_value=1  m_nominal_unit=kg  T_specify=on  T_priority=High  T=vehicleThermal.cabin_T_init K  T_nominal_specify=off  T_nominal_value=cabin_T_init  T_nominal_unit=degC  Q_specify=off  Q_priority=None  Q=0 W  Q_nominal_specify=off  Q_nominal_value=1  Q_nominal_unit=W
  PTC Air Volume : fl_lib/Moist Air/Elements/Constant Volume Chamber (MA)  volume=0.001 m^3  num_ports=foundation.enum.num_ports.two  area_A=HVAC.cabin_duct_area m^2  area_B=HVAC.cabin_duct_area m^2  area_C=0.01 m^2  area_D=0.01 m^2  RH_ws=1  time_constant_cond=1e-3 s  time_constant_evap=1e-3 s  fraction_entrained=1  moisture_trace_gas_source=foundation.enum.moisture_trace_gas_source.none  moisture_source_spec=foundation.enum.MoistureSourceSpec.WaterVapor  vapor_from_liquid=false  moisture_mass_flow=0 kg/s  moisture_temperature_spec=foundation.enum.temperature_spec.atmospheric  moisture_temperature=293.15 K  trace_gas_mass_flow=0 kg/s  trace_gas_temperature_spec=foundation.enum.temperature_spec.atmospheric  trace_gas_temperature=293.15 K  p_init=vehicleThermal.cabin_p_init MPa  p_init_priority=foundation.enum.Priority.High  T_init=vehicleThermal.cabin_T_init K  T_init_priority=foundation.enum.Priority.High  humidity_spec=foundation.enum.HumiditySpec.RelativeHumidity  RH_init=vehicleThermal.cabin_RH_init  RH_init_priority=foundation.enum.Priority.High  x_w_init=0  x_w_init_priority=foundation.enum.Priority.None  y_w_init=0  y_w_init_priority=foundation.enum.Priority.None  HR_init=0  HR_init_priority=foundation.enum.Priority.None  Tw_init=287 K  Tw_init_priority=foundation.enum.Priority.High  trace_gas_spec=foundation.enum.trace_gas_spec.mass_fraction  x_g_init=0  x_g_init_priority=foundation.enum.Priority.High  y_g_init=0  y_g_init_priority=foundation.enum.Priority.None  r_d_init=0  r_d_init_priority=foundation.enum.Priority.High
      settings: InternalSimscapePortConfiguration="{\"Bottom\":[],\"Left\":[{\"id\":\"A\",\"label\":\"A\",\"type\":\"foundation.moist_air.moist_air\"},{\"id\":\"B\",\"label\":\"B\",\"type\":\"foundation.moist_air.moist_air\"}],\"Right\":[{\"id\":\"W\",\"label\":\"W\",\"type\":\"output\"},{\"id\":\"F\",\"label\":\"F\",\"type\":\"output\"},{\"id\":\"H\",\"label\":\"H\",\"type\":\"foundation.thermal.thermal\"}],\"Top\":[]}"
  Pressure & Temperature Sensor (MA) : fl_lib/Moist Air/Sensors/Pressure & Temperature Sensor (MA)  reference=foundation.enum.MeasurementReference.difference  pressure=true  pressure_spec=foundation.enum.PressureMeasementSpec.Absolute  temperature=true
      settings: InternalSimscapePortConfiguration="{\"Bottom\":[{\"id\":\"T\",\"label\":\"T\",\"type\":\"output\"}],\"Left\":[{\"id\":\"A\",\"label\":\"A\",\"type\":\"foundation.moist_air.moist_air\"}],\"Right\":[{\"id\":\"B\",\"label\":\"B\",\"type\":\"foundation.moist_air.moist_air\"},{\"id\":\"P\",\"label\":\"P\",\"type\":\"output\"}],\"Top\":[]}"
  Simulink-PS Converter1 : nesl_utility/Simulink-PS Converter  PhysicalDomain=network_engine_domain  SubClassName=ps_input  LeftPortType=input  RightPortType=output  PseudoPeriodic=off  Frequencies=[]  NoiseDistribution=none  NoiseParameters=[]  Unit=W  AffineConversion=off  FilteringAndDerivatives=provide  SimscapeFilterOrder=1  InputFilterTimeConstant=0.001  UdotUserProvided=0
  Solver Configuration : nesl_utility/Solver Configuration  PhysicalDomain=network_engine_domain  SubClassName=solver  LeftPortType=input  RightPortType=generic  Tones=[]  Harmonics=[]  SimulateNoise=off  Profile=off  UseLocalSampling=off  EnableSwitchedLinearOptims=on  FrequencyDomain=off  UseCCode=off  RelTol=0.001  AbsTol=1e-06  MinStep=1e-09  ToWorkspace=off  RevertToSquareIcSolve=off  NumHomotopyIterations=100  PhasorMode=off  PhasorModeNumHarmonics=1  ConsistencySolver=NEWTON_XTOL_AFTER_FTOL  IndexReductionMethod=DerivativeReplacement  DoDC=off  ResidualTolerance=1e-9  ConsistencyTolSource=GLOBAL  ConsistencyAbsTol=0.001  ConsistencyRelTol=0.001  ConsistencyTolFactor=0.001  UseLocalSolver=off  LocalSolverChoice=NE_BACKWARD_EULER_ADVANCER  ResolveIndetEquations=on  FunctionEvalNumThread=1  LocalSolverSampleTime=0.1  DoFixedCost=off  MaxNonlinIter=3  MaxModeIter=2  ComputeImpulses=off  ImpulseIterations=2  LinearAlgebra=auto  LinearAlgebraNumThread=0  EquationFormulation=NE_TIME_EF  DelaysMemoryBudget=1024  AutomaticFiltering=on  FilteringTimeConstant=0.001  PartitionStorageMethod=AS_NEEDED  PartitionMemoryBudget=1024  PartitionMethod=FAST  MultibodyUseLocalSolver=off  MultibodyLocalSolverChoice=ODE1  MultibodyLocalSolverSampleTime=0.001
  Thermal Reference : fl_lib/Thermal/Thermal Elements/Thermal Reference
  B : PMIOPort  Side=Left
  A : PMIOPort  Port=2  Side=Right
  T : Outport
  wires:
  PS-Simulink Converter/1 -> T/1
  cmd/1 -> Simulink-PS Converter1/1
  connections:
  A/RConn1 -- Flow Resistance (MA)/LConn1
  Flow Resistance (MA)1/RConn1 -- B/RConn1 -- Pressure & Temperature Sensor (MA)/LConn1
  Pressure & Temperature Sensor (MA)/RConn3 -- PS-Simulink Converter/LConn1
  Absolute Reference (MA)/LConn1 -- Pressure & Temperature Sensor (MA)/RConn1
  PTC Air Volume/RConn3 -- Convective Heat Transfer/RConn1
  PTC Air Volume/LConn2 -- Flow Resistance (MA)1/LConn1
  Flow Resistance (MA)/RConn1 -- PTC Air Volume/LConn1
  Controlled Heat Flow Rate Source/RConn2 -- Solver Configuration/RConn1 -- Thermal Reference/LConn1
  Simulink-PS Converter1/RConn1 -- Controlled Heat Flow Rate Source/RConn1
  Controlled Heat Flow Rate Source/LConn1 -- PTC Thermal Mass/LConn1 -- Convective Heat Transfer/LConn1

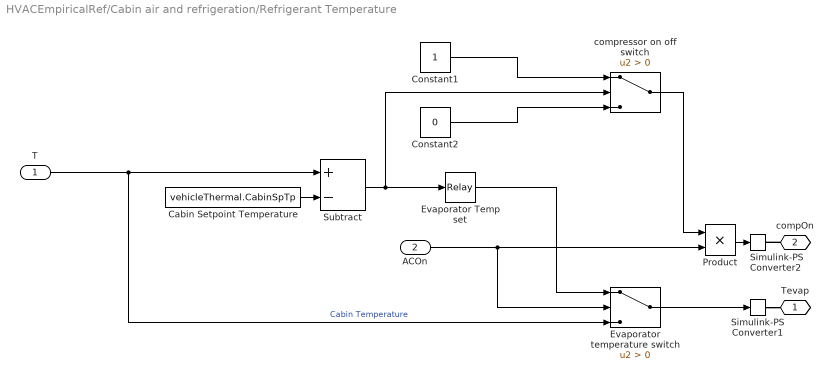
== system HVACEmpiricalRef/Cabin air and refrigeration/Refrigerant Temperature ==
  T : Inport
  ACOn : Inport  Port=2
  Cabin Setpoint Temperature : Constant  Value=vehicleThermal.CabinSpTp
  Constant1 : Constant
  Constant2 : Constant  Value=0
  Evaporator Temp set : Relay  OnSwitchValue=1  OffSwitchValue=-0.1  OnOutputValue=RefTemp  OffOutputValue=vehicleThermal.ambient  ZeroCross=off
  "Evaporator temperature switch " : Switch  Criteria=u2 > Threshold  SaturateOnIntegerOverflow=off  InputSameDT=off
  Product : Product
  Simulink-PS Converter1 : nesl_utility/Simulink-PS Converter  PhysicalDomain=network_engine_domain  SubClassName=ps_input  LeftPortType=input  RightPortType=output  PseudoPeriodic=off  Frequencies=[]  NoiseDistribution=none  NoiseParameters=[]  Unit=K  AffineConversion=off  FilteringAndDerivatives=filter  SimscapeFilterOrder=1  InputFilterTimeConstant=1  UdotUserProvided=0
  Simulink-PS Converter2 : nesl_utility/Simulink-PS Converter  PhysicalDomain=network_engine_domain  SubClassName=ps_input  LeftPortType=input  RightPortType=output  PseudoPeriodic=off  Frequencies=[]  NoiseDistribution=none  NoiseParameters=[]  Unit=1  AffineConversion=off  FilteringAndDerivatives=filter  SimscapeFilterOrder=1  InputFilterTimeConstant=1  UdotUserProvided=0
  Subtract : Sum  Inputs=+-
  compressor on off switch : Switch  Criteria=u2 > Threshold  SaturateOnIntegerOverflow=off  InputSameDT=off
  Tevap : PMIOPort  Side=Right
  compOn : PMIOPort  Port=2  Side=Right
  wires:
  Product/1 -> Simulink-PS Converter2/1
  compressor on off switch/1 -> Product/1
  Constant2/1 -> compressor on off switch/3
  Constant1/1 -> compressor on off switch/1
  "Evaporator temperature switch "/1 -> Simulink-PS Converter1/1
  Evaporator Temp set/1 -> "Evaporator temperature switch "/1
  Subtract/1 -> compressor on off switch/2, Evaporator Temp set/1
  ACOn/1 -> Product/2, "Evaporator temperature switch "/2
  Cabin Setpoint Temperature/1 -> Subtract/2
  T/1 -> "Evaporator temperature switch "/3, Subtract/1  "Cabin Temperature"
  connections:
  compOn/RConn1 -- Simulink-PS Converter2/RConn1
  Simulink-PS Converter1/RConn1 -- Tevap/RConn1

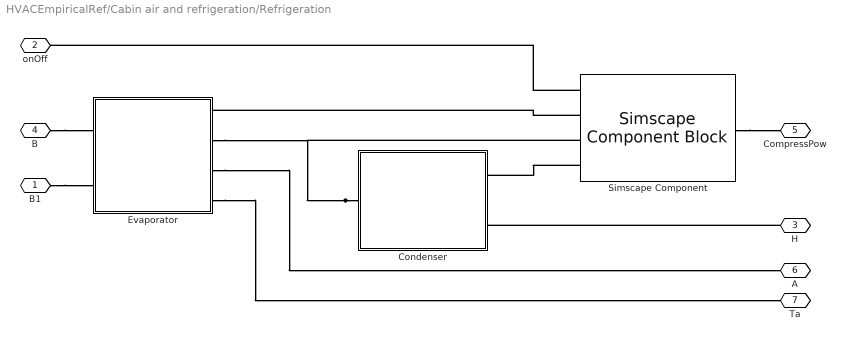
== system HVACEmpiricalRef/Cabin air and refrigeration/Refrigeration ==
  Condenser : Subsystem
  Evaporator : Subsystem
  Simscape Component : SimscapeComponentBlock  SourceFile=compressorPower  ComponentPath=compressorPower  ComponentVariants="[\"compressorPower\"]"  ComponentVariantNames="[\"compressorPower\"]"  ClassName=compressorPower  SchemaVersion=1  systemEfficiency=0.7
      settings: CopyFcn=simscape.engine.sli.internal.componentblockcallback(gcbh,'COPY')  PreCopyFcn=simscape.engine.sli.internal.componentblockcallback(gcbh,'PRECOPY')  PreDeleteFcn=simscape.engine.sli.internal.componentblockcallback(gcbh,'PREDELETE')  InternalSimscapePortConfiguration="{\"Bottom\":[],\"Left\":[{\"id\":\"compOn\",\"label\":\"compOn\",\"type\":\"input\"},{\"id\":\"Tevap\",\"label\":\"Tevap\",\"type\":\"input\"},{\"id\":\"Qcond\",\"label\":\"Qcond\",\"type\":\"input\"},{\"id\":\"Tcond\",\"label\":\"Tcond\",\"type\":\"input\"}],\"Right\":[{\"id\":\"compressPow\",\"label\":\"compressPow\",\"type\":\"output\"}],\"Top\":[]}"
      mask Type: This block computes theoretical compressor power.
  B1 : PMIOPort  Side=Left
  onOff : PMIOPort  Port=2  Side=Left
  H : PMIOPort  Port=3  Side=Left
  B : PMIOPort  Port=4  Side=Right
  CompressPow : PMIOPort  Port=5  Side=Right
  A : PMIOPort  Port=6  Side=Right
  Ta : PMIOPort  Port=7  Side=Right
  connections:
  Simscape Component/LConn1 -- onOff/RConn1
  Simscape Component/LConn2 -- Evaporator/RConn1
  Simscape Component/LConn4 -- Condenser/RConn1
  Simscape Component/RConn1 -- CompressPow/RConn1
  Evaporator/RConn3 -- A/RConn1
  B/RConn1 -- Evaporator/LConn1
  Condenser/LConn1 -- Simscape Component/LConn3 -- Evaporator/RConn2
  H/RConn1 -- Condenser/RConn2
  B1/RConn1 -- Evaporator/LConn2
  Evaporator/RConn4 -- Ta/RConn1
